simulink subsystem "Motor_subsystem"  (R2020a)
settings: Solver=VariableStepAuto  StartTime=0.0  StopTime=10.0  RelTol=1e-3
values from neighbouring files (symbols this model uses):
  Jm = 0.05    [Servo_motor.mat]
  Kb = 0.1    [Servo_motor.mat]
  Ki = 5    [Servo_motor.mat]
  L = 0.005    [Servo_motor.mat]
  R = 1    [Servo_motor.mat]
settings Model: Creator=Haier  LastModifiedBy=Haier

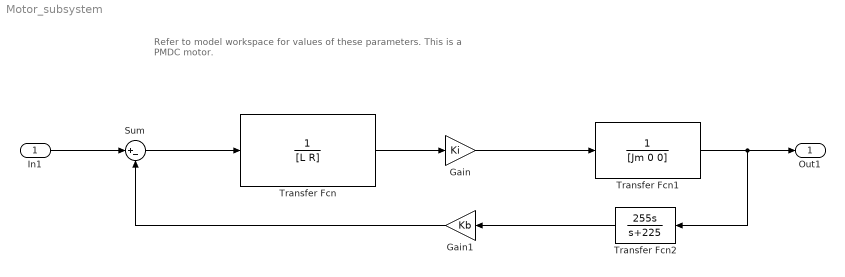
== system Motor_subsystem ==
  note: Refer to model workspace for values of these
      | parameters. This is a PMDC motor.
  In1 : Inport
  Gain : Gain  Gain=Ki
  Gain1 : Gain  Gain=Kb
  Sum : Sum  Inputs=|+-
  Transfer Fcn : TransferFcn  Denominator=[L R]
  Transfer Fcn1 : TransferFcn  Denominator=[Jm 0 0]
  Transfer Fcn2 : TransferFcn  Numerator=[255 0]  Denominator=[1 225]
  Out1 : Outport
  wires:
  Gain1/1 -> Sum/2
  Transfer Fcn1/1 -> Transfer Fcn2/1, Out1/1
  Transfer Fcn2/1 -> Gain1/1
  Gain/1 -> Transfer Fcn1/1
  Sum/1 -> Transfer Fcn/1
  Transfer Fcn/1 -> Gain/1
  In1/1 -> Sum/1
